simulink model "FAS_Kreuzungswarner_Simulation_V1"  (R2024b)
settings: Solver=FixedStepAuto  StartTime=0.0  StopTime=stoptime  FixedStep=sampletime  RelTol=1e-3
InitFcn:
  | if ~evalin('base', 'exist(''Auswertungsflag'', ''var'')') || evalin('base', 'Auswertungsflag.Value == 0')
  |     Parameterskript;
  |     run('StartGUI');  % explizit ausführen (nicht blockierend!)
  | end
values from neighbouring files (symbols this model uses):
  mEGO = str2double(massEGOInput.String)    [StartGUI.m]
  mFZG = str2double(massFZGInput.String)    [StartGUI.m]
  OeffnungswinkelA = str2double(angleInputA.String)    [StartGUI.m]
  OeffnungswinkelB = Simulink.Parameter    [Auswertung.m]    (also in StartGUI.m = str2double(angleInputB.String))
  P_EGO = str2double(powerEGOInput.String)    [StartGUI.m]
  P_FZG = str2double(powerFZGInput.String)    [StartGUI.m]
  ReichweiteA = str2double(rangeInputA.String)    [StartGUI.m]
  ReichweiteB = str2double(rangeInputB.String)    [StartGUI.m]
  SensorA = sensor1Dropdown.Value    [StartGUI.m]
  SensorB = sensor2Dropdown.Value    [StartGUI.m]
  startPositionEGO = str2double(posEGOInput.String)    [StartGUI.m]
  startPositionFzg = str2double(posFzgInput.String)    [StartGUI.m]
  v_EGO = str2double(velEGOInput.String)    [StartGUI.m]
  v_FZG = str2double(velFZGInput.String)    [StartGUI.m]
  Wetter = weatherDropdown.Value    [StartGUI.m]
  zweitesFzgSwitch = str2double(zweitesFzgInput.String)    [StartGUI.m]
undefined symbols (not defined in the file or in its folder): Airbagzeit, Ausloesezeit, b, dt, g, Haltezeit, l, munass, muschnee, mutrocken, rad_b, rad_l, reifen_dx, reifen_dy, SensorSwitch, startPositionFzg2, xFZG, yEGO
(part 1 of 3)
settings Model: Creator=panic  LastModifiedBy=flori
settings DataIOCC: SaveFormat=StructureWithTime

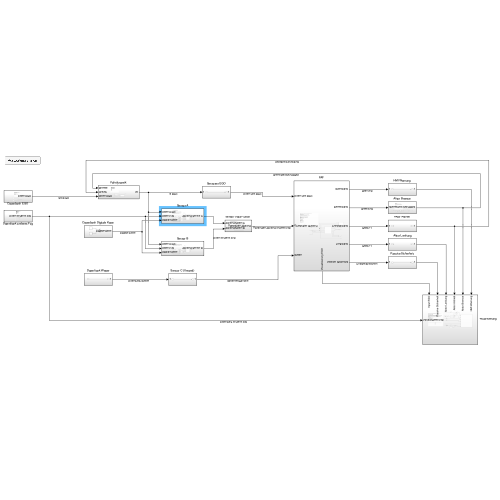
[thumbnail: Simulink's stored preview of the top-level diagram]
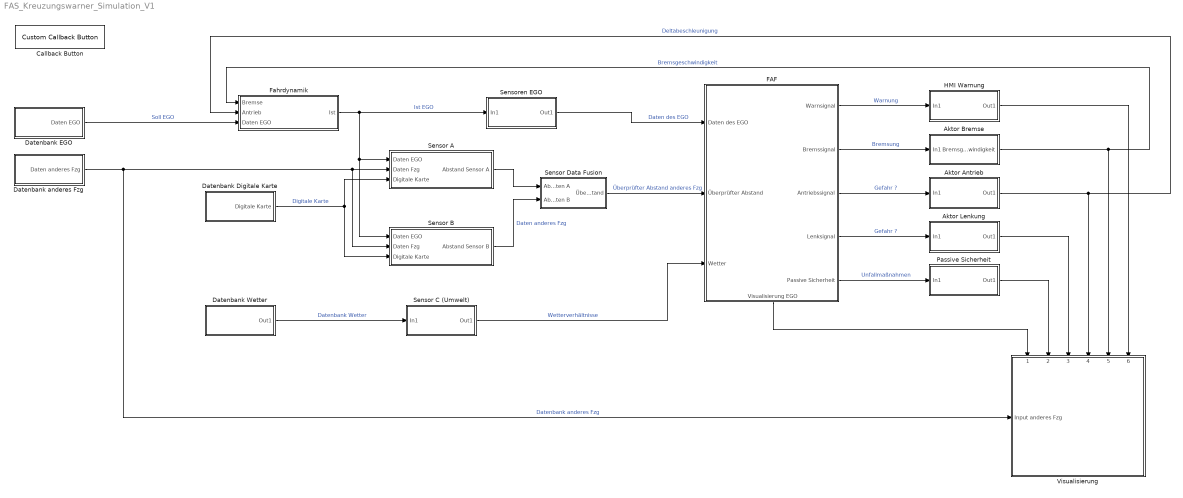
== system FAS_Kreuzungswarner_Simulation_V1 ==
  " Aktor Lenkung" : Subsystem
  Aktor Antrieb : Subsystem
  Aktor Bremse : Subsystem
  Callback Button : CustomCallbackButton  Configuration="{\"components\":[{\"name\":\"BackgroundImageComponent\",\"settings\":{\"image\":{\"size\":[0,0],\"src\":\"default\",\"srcOrientation\":\"Right\"},\"position\":[0,0,1,1]}},{\"name\":\"ButtonStateComponent\",\"settings\":{\"buttonType\":\"momentary\",\"clickFcn\":\"clear all\\nclc\\nassignin('base','Auswertungsbutton',makeParam(1));\\nStartGUI\",\"onValue\":1,\"position\":[0,0,1,1],\"pressDelay\":\"500\",\"pressFcn\":\"\",\"repeatInterval\":\"0\",\"states\":[{\"horizontalAlignment\":\"center\",\"image\":{\"position\":[0,0,1,1],\"size\":[1,1],\"src\":\"default\",\"srcOrientation\":\"Right\"},\"label\":{\"color\":[0,0,0],\"icon\":{\"size\":[0,0],\"src\":\"default\",\"srcOrientation\":\"Right\"},\"iconOffset\":0,\"iconPlacement\":\"left\",\"opacity\":1,\"show\":true,\"text\":{\"content\":\"Auswertung starten\",\"font\":\"Helvetica\"}},\"labelOffset\":[0,0],\"verticalAlignment\":\"middle\"},{\"horizontalAlignment\":\"center\",\"image\":{\"position\":[0,0,1,1],\"size\":[1,1],\"src\":\"default\",\"srcOrientation\":\"Right\"},\"label\":{\"color\":[0.01176470588,0.01176470588,0.01176470588,1],\"icon\":{\"size\":[0,0],\"src\":\"default\",\"srcOrientation\":\"Right\"},\"iconOffset\":0,\"iconPlacement\":\"left\",\"opacity\":1,\"show\":true,\"text\":{\"content\":\"Auswertung starten\",\"font\":\"Helvetica\"}},\"labelOffset\":[0,0],\"verticalAlignment\":\"middle\"},{\"horizontalAlignment\":\"center\",\"image\":{\"position\":[0,0,1,1],\"size\":[1,1],\"src\":\"default\",\"srcOrientation\":\"Right\"},\"label\":{\"color\":[0.01176470588,0.01176470588,0.01176470588,1],\"icon\":{\"size\":[0,0],\"src\":\"default\",\"srcOrientation\":\"Right\"},\"iconOffset\":0,\"iconPlacement\":\"left\",\"opacity\":1,\"show\":true,\"text\":{\"content\":\"Auswertung starten\",\"font\":\"Helvetica\"}},\"labelOffset\":[0,0],\"verticalAlignment\":\"middle\"},{\"horizontalAlignment\":\"center\",\"image\":{\"position\":[0,0,1,1],\"size\":[1,1],\"src\":\"default\",\"srcOrientation\":\"Right\"},\"label\":{\"color\":[0.01176470588,0.01176470588,0.01176470588,1],\"icon\":{\"size\":[0,0],\"src\":\"default\",\"srcOrientation\":\"Right\"},\"iconOffset\":0,\"iconPlacement\":\"left\",\"opacity\":1,\"show\":true,\"text\":{\"content\":\"Auswertung starten\",\"font\":\"Helvetica\"}},\"labelOffset\":[0,0],\"verticalAlignment\":\"middle\"}]}},{\"name\":\"ForegroundImageComponent\",\"settings\":{\"image\":{\"size\":[0,0],\"src\":\"default\",\"srcOrientation\":\"Right\"},\"isForeground\":1,\"position\":[0,0,1,1]}}],\"settings\":{\"BindingType\":\"standalone\",\"backgroundColor\":[244,244,244,1],\"backgroundOffset\":0.2,\"backgroundOpacity\":1,\"fixedAspectRatio\":\"off\",\"foregroundColor\":[0.01176470588,0.01176470588,0.01176470588,1],\"migratedFromLegacy\":true,\"useBackgroundColor\":true,\"variant\":\"callback\",\"version\":\"R2023a\"},\"type\":\"Button\"}"  CustomBackgroundColor="{\"color\":[0.9568627451,0.9568627451,0.9568627451],\"show\":true}"
  Datenbank Digitale Karte : Subsystem
  Datenbank EGO : Subsystem
  Datenbank Wetter : Subsystem
  Datenbank anderes Fzg : Subsystem
  FAF : Subsystem
      settings: PortSchema="{\"entries\":[{\"content\":{\"sides\":[{\"content\":{\"connectorIds\":[\"In1\",\"In2\",\"In3\"]},\"type\":\"ConnectorPlacement.EquallySpacedRectSide\",\"uuid\":\"e9873d16-4c3b-480f-9547-2fedddc84fa2\"},{\"content\":{\"connectorIds\":[\"Out1\",\"Out2\",\"Out3\",\"Out4\",\"Out5\"],\"side\":\"RIGHT\"},\"type\":\"ConnectorPlacement.EquallySpacedRectSide\",\"uuid\":\"f34f386d-1ebd-46c0-87cc-6cf8d85cbe5c\"},{\"content\":{\"side\":\"TOP\"},\"type\":\"ConnectorPlacement.EquallySpacedRectSide\",\"uuid\":\"dae2a922-0ae9-4030-aebb-c1b1f64935ac\"},{\"content\":{\"connectorIds\":[\"Out6\"],\"side\":\"BOTTOM\"},\"type\":\"ConnectorPlacement.EquallySpacedRectSide\",\"uuid\":\"92c182dc-0911-4a88-8c5f-7399a74ff050\"}]},\"type\":\"ConnectorPlacement.EquallySpacedConnector\",\"uuid\":\"9c5e93a9-4ab8-4391-bbf4-9015a537a4fe\"}],\"packageUris\":[\"http://schema.mathworks.com/mf0/Connector/R2020b\"],\"version\":\"1.0\"}"
  Fahrdynamik : Subsystem
  HMI Warnung : Subsystem
  Passive Sicherheit : Subsystem
  Sensor A : Subsystem
  Sensor B : Subsystem
  Sensor C (Umwelt) : Subsystem
  "Sensor Data Fusion " : Subsystem
  Sensoren EGO : Subsystem
  Visualisierung : Subsystem
      settings: PortSchema="{\"entries\":[{\"content\":{\"sides\":[{\"content\":{\"connectorIds\":[\"In1\",\"In2\",\"In3\",\"In4\",\"In5\",\"In6\"]},\"type\":\"ConnectorPlacement.EquallySpacedRectSide\",\"uuid\":\"dd165e45-7e24-4222-b079-fc0a14401503\"},{\"content\":{\"side\":\"RIGHT\"},\"type\":\"ConnectorPlacement.EquallySpacedRectSide\",\"uuid\":\"187c38cf-364e-4c00-8f01-04e514044ebb\"},{\"content\":{\"connectorIds\":[\"In7\"],\"side\":\"TOP\"},\"type\":\"ConnectorPlacement.EquallySpacedRectSide\",\"uuid\":\"80aec09e-8245-4401-9644-d123aeedc7c7\"}]},\"type\":\"ConnectorPlacement.EquallySpacedConnector\",\"uuid\":\"48ae2ddf-e251-4d97-a6a7-fcee22a63fde\"}],\"packageUris\":[\"http://schema.mathworks.com/mf0/Connector/R2020b\"],\"version\":\"1.0\"}"
  wires:
  Fahrdynamik/1(Ist) -> Sensor B/1(Daten EGO), Sensor A/1(Daten EGO), Sensoren EGO/1(In1)  "Ist EGO"
  Sensoren EGO/1(Out1) -> FAF/1(Daten des EGO)  "Daten des EGO"
  Sensor C (Umwelt)/1(Out1) -> FAF/3(Wetter)  "Wetterverhältnisse"
  FAF/3(Antriebssignal) -> Aktor Antrieb/1(In1)  "Gefahr ?"
  FAF/2(Bremssignal) -> Aktor Bremse/1(In1)  "Bremsung"
  FAF/1(Warnsignal) -> HMI Warnung/1(In1)  "Warnung"
  FAF/4(Lenksignal) -> " Aktor Lenkung"/1(In1)  "Gefahr ?"
  FAF/5(Passive Sicherheit) -> Passive Sicherheit/1(In1)  "Unfallmaßnahmen"
  FAF/6(Visualisierung EGO) -> Visualisierung/1(Input EGO)
  Passive Sicherheit/1(Out1) -> Visualisierung/2(Passive Sicherheit)
  " Aktor Lenkung"/1(Out1) -> Visualisierung/3(Aktor Lenkung)
  Aktor Antrieb/1(Out1) -> Visualisierung/4(Aktor Antrieb), Fahrdynamik/2(Antrieb)  "Deltabeschleunigung"
  Aktor Bremse/1(Bremsgeschwindigkeit) -> Visualisierung/5(Aktor Bremse), Fahrdynamik/1(Bremse)  "Bremsgeschwindigkeit"
  HMI Warnung/1(Out1) -> Visualisierung/6(HMI Warnung)
  Datenbank Digitale Karte/1(Digitale Karte) -> Sensor B/3(Digitale Karte), Sensor A/3(Digitale Karte)  "Digitale Karte"
  Datenbank EGO/1(Daten EGO) -> Fahrdynamik/3(Daten EGO)  "Soll EGO"
  Datenbank anderes Fzg/1(Daten anderes Fzg) -> Sensor B/2(Daten Fzg), Sensor A/2(Daten Fzg), Visualisierung/7(Input anderes Fzg)  "Datenbank anderes Fzg"
  Sensor B/1(Abstand Sensor B) -> "Sensor Data Fusion "/2(Abstandsdaten B)  "Daten anderes Fzg"
  Sensor A/1(Abstand Sensor A) -> "Sensor Data Fusion "/1(Abstandsdaten A)
  "Sensor Data Fusion "/1(Überprüfter Abstand) -> FAF/2(Überprüfter Abstand)  "Überprüfter Abstand anderes Fzg"
  Datenbank Wetter/1(Out1) -> Sensor C (Umwelt)/1(In1)  "Datenbank Wetter"

== system FAS_Kreuzungswarner_Simulation_V1/ Aktor Lenkung ==
  In1 : Inport
  Out1 : Outport

== system FAS_Kreuzungswarner_Simulation_V1/Aktor Antrieb ==
  In1 : Inport
  Out1 : Outport

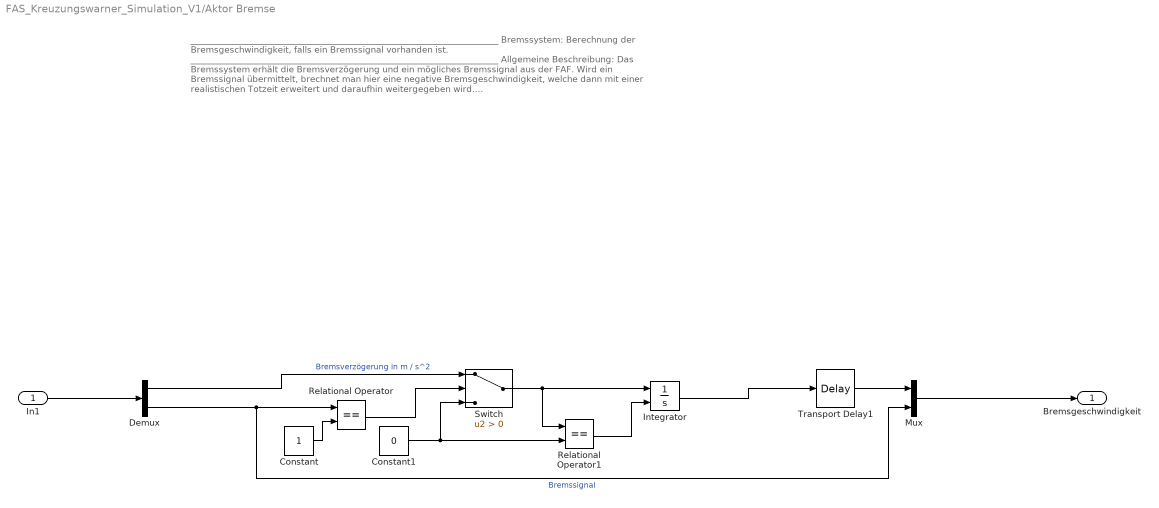
== system FAS_Kreuzungswarner_Simulation_V1/Aktor Bremse ==
  note: _______________________________________________________________________
      | Bremssystem:
      |
      | Berechnung der Bremsgeschwindigkeit, falls ein Bremssignal vorhanden ist.
      | _______________________________________________________________________
      | Allgemeine Beschreibung:
      |
      | Das Bremssystem erhält die Bremsverzögerung und ein mögliches Bremssignal aus
      | der FAF.
      | Wird ein Bremssignal übermittelt, brechnet man hier eine negative Bremsgeschwindigkeit,
      | welche dann mit einer realistischen Totzeit erweitert und daraufhin weitergegeben wird.
      | _______________________________________________________________________
      | Inputs:
      |
      | Das Bremssystem hat zwei Inputs:
      |
      | - Bremsverzögerung [m/s^2]
      | - Bremssignal als 0/1 Signal
      |
      | Outputs:
      |
      | - Berechnete Bremsgeschwindigkeit [m/s]
      | _______________________________________________________________________
  In1 : Inport
  Constant : Constant
  Constant1 : Constant  Value=0
  Demux : Demux  Outputs=2
  Integrator : Integrator  ExternalReset=level
  Mux : Mux  Inputs=2
  Relational Operator : RelationalOperator  Operator===  OutDataTypeStr=boolean  RndMeth=Simplest  InputSameDT=off
  Relational Operator1 : RelationalOperator  Operator===  OutDataTypeStr=boolean  RndMeth=Simplest  InputSameDT=off
  Switch : Switch  Criteria=u2 > Threshold  SaturateOnIntegerOverflow=off  InputSameDT=off
  Transport Delay1 : TransportDelay  DelayTime=0.3
  Bremsgeschwindigkeit : Outport
  wires:
  In1/1 -> Demux/1
  Demux/1 -> Switch/1  "Bremsverzögerung in m / s^2"
  Demux/2 -> Relational Operator/1, Mux/2  "Bremssignal"
  Mux/1 -> Bremsgeschwindigkeit/1
  Constant/1 -> Relational Operator/2
  Relational Operator/1 -> Switch/2
  Relational Operator1/1 -> Integrator/2
  Integrator/1 -> Transport Delay1/1
  Constant1/1 -> Relational Operator1/2, Switch/3
  Switch/1 -> Integrator/1, Relational Operator1/1
  Transport Delay1/1 -> Mux/1

== system FAS_Kreuzungswarner_Simulation_V1/Datenbank Digitale Karte ==
  Mux : Mux  Inputs=2
  xPos Kreuzung : Constant  Value=0
  yPos Kreuzung1 : Constant  Value=0
  Digitale Karte : Outport
  wires:
  Mux/1 -> Digitale Karte/1
  yPos Kreuzung1/1 -> Mux/2
  xPos Kreuzung/1 -> Mux/1

== system FAS_Kreuzungswarner_Simulation_V1/Datenbank EGO ==
  note: _______________________________________________________________________
      | Datenbank EGO:
      |
      | Vorgabe aller Werte die das EGO-Fahrzeug beinhaltet / benötigt.
      | _______________________________________________________________________
      | Allgemeine Beschreibung:
      |
      | Die Werte die das EGO-Fahrzeug erhält werden über das Parameterskript initialisiert und
      | dann über die Eingabe in der GUI angepasst. Daraufhin werden Sie hier in die
      | unterschieldichen Blöcke gespeichert.
      | Die Geschwindigkeit wird nach der Eingabe in m/s umgerechnet.
      | _______________________________________________________________________
      | Inputs:
      |
      | Die Datenbank des EGOs beinhaltet drei Werte:
      |
      | - Motorleistung_EGO [kW]
      | - Fahrzeugmasse_EGO [kg]
      | - Geschwindikeit_EGO [km/h]
      |
      | Outputs:
      |
      | Diese Werte werden dann an die Fahrdynamik weitergeleitet.
      | ______________________________________________________________________
  Fahrzeugmasse in kg : Constant  Value=mEGO
  Gain : Gain  Gain=1/3.6
  Geschwindigkeit km/h : Constant  Value=v_EGO
  Motorleistung in kW : Constant  Value=P_EGO
  Mux : Mux  Inputs=3
  Daten EGO : Outport
  wires:
  Fahrzeugmasse in kg/1 -> Mux/2
  Motorleistung in kW/1 -> Mux/1
  Mux/1 -> Daten EGO/1
  Geschwindigkeit km/h/1 -> Gain/1
  Gain/1 -> Mux/3  "GeschwindigkeitEGO in m/s"

== system FAS_Kreuzungswarner_Simulation_V1/Datenbank Wetter ==
  Regen : Constant  Value=Wetter
  Out1 : Outport
  wires:
  Regen/1 -> Out1/1

== system FAS_Kreuzungswarner_Simulation_V1/Datenbank anderes Fzg ==
  note: _______________________________________________________________________
      | Datenbank anderes Fahrzeug:
      |
      | Vorgabe aller Werte die die anderen Fahrzeuge beinhalten / benötigen.
      | _______________________________________________________________________
      | Allgemeine Beschreibung:
      |
      | Die Werte die das andere Fahrzeug erhält werden über das Parameterskript initialisiert und
      | dann über die Eingabe in der GUI angepasst. Daraufhin werden Sie hier in die
      | unterschiedlichen Blöcke gespeichert.
      | Zusätzlich werden auch hier nochmals die Werte des EGO-Fahrzeugs verwendet (diese werden für das Szenario mit dem vorrausfahrenden Fahrzeug (zweites FZG) benötigt).
      | Die Geschwindigkeiten werden nach der Eingabe in m/s umgerechnet.
      | _______________________________________________________________________
      | Inputs:
      |
      | Die Datenbank der anderen Fahrzeuge beinhaltet folgende Werte:
      |
      | - Motorleistung des anderen Fahrzeugs [kW]
      | - Fahrzeugmasse des anderen Fahrzeugs [kg]
      | - Geschwindigkeit des anderen Fahrzeugs [km/h]
      |
      | - Motorleistung_EGO [kW]
      | - Fahrzeugmasse_EGO [kg]
      | - Geschwindikeit_EGO [km/h]
      |
      | Outputs:
      |
      | Diese Werte werden dann teilweise an die Sensoren (A und B), aber auch an die
      | Visualisierung weitergeleitet.
      | ______________________________________________________________________
  Fahrzeugmasse in kg : Constant  Value=mFZG
  Fahrzeugmasse in kg1 : Constant  Value=mEGO
  Gain : Gain  Gain=1/3.6
  Gain1 : Gain  Gain=1/3.6
  Geschwindigkeit km/h : Constant  Value=v_FZG
  Geschwindigkeit km/h1 : Constant  Value=v_EGO
  Motorleistung in kW : Constant  Value=P_FZG
  Motorleistung in kW1 : Constant  Value=P_EGO
  Mux : Mux  Inputs=6
  Daten anderes Fzg : Outport
  wires:
  Fahrzeugmasse in kg/1 -> Mux/2
  Motorleistung in kW/1 -> Mux/1
  Geschwindigkeit km/h/1 -> Gain/1
  Mux/1 -> Daten anderes Fzg/1
  Gain/1 -> Mux/3
  Geschwindigkeit km/h1/1 -> Gain1/1
  Fahrzeugmasse in kg1/1 -> Mux/5
  Gain1/1 -> Mux/6
  Motorleistung in kW1/1 -> Mux/4

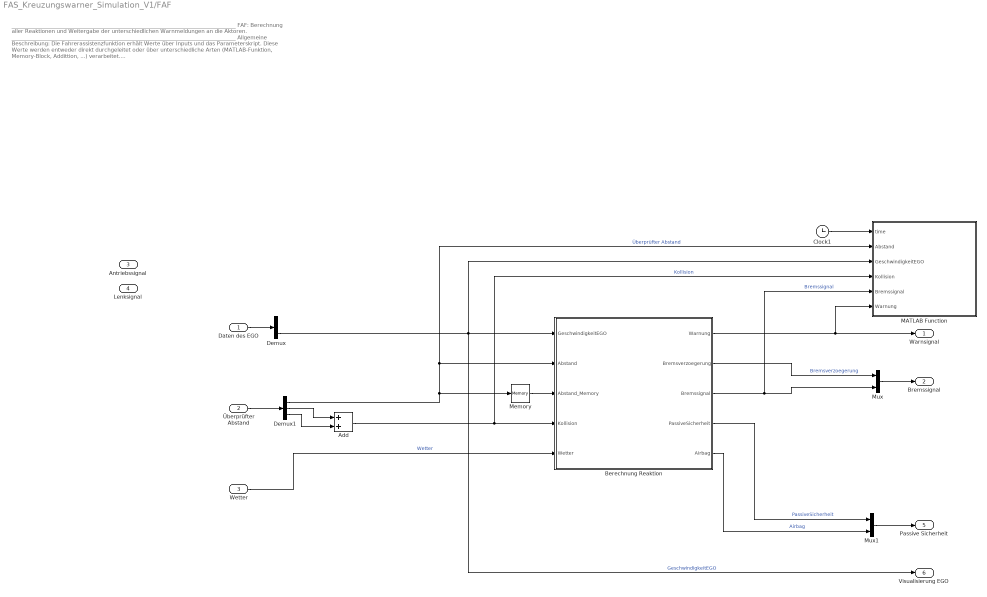
== system FAS_Kreuzungswarner_Simulation_V1/FAF ==
  note: ____________________________________________________________________________________
      | FAF:
      |
      | Berechnung aller Reaktionen und Weitergabe der unterschiedlichen Warnmeldungen an die Aktoren.
      | ____________________________________________________________________________________
      | Allgemeine Beschreibung:
      |
      | Die Fahrerassistenzfunktion erhält Werte über Inputs und das Parameterskript.
      | Diese Werte werden entweder direkt durchgeleitet oder über unterschiedliche Arten
      | (MATLAB-Funktion, Memory-Block, Addittion, ...) verarbeitet.
      | ____________________________________________________________________________________
      | Inputs:
      |
      | Die FAF beinhaltet aktive, während der Simulation veränderliche, Inputs:
      |
      | - Geschwindikeit_EGO [m/s]
      | - Abstand [m]
      | - Abstand_Memory [m] (= Abstand des vorherigen Simulationsschritts)
      | - Kollision als 0/1 Signal (wenn Kollision = 1, Fahrzeuge treffen sich)
      | - Wetter (Trocken, Regen und Schnee)
      |
      | Outputs:
      |
      | - Warnung als 0/1 Signal
      | - Bremsverzögerung in m/s^2
      | - Bremssignal als 0/1 Signal
      | - Passive Sicherheit als 0/1 Signal
      | - Airbag als 0/1 Signal
      |
      | Reserve
      | - Antriebssignal für spätere Projekte
      |
      | - Lenksignal für spätere Projekte
      |
      | _______________________________________________________________________
  Daten des EGO : Inport
  Überprüfter Abstand : Inport  Port=2
  Wetter : Inport  Port=3
  Add : Sum
  Berechnung Reaktion : MATLAB Function  TreatAsAtomicUnit=on
  Clock1 : Clock
  Demux : Demux  Outputs=3
  Demux1 : Demux  Outputs=3
  MATLAB Function : MATLAB Function  TreatAsAtomicUnit=on  SystemSampleTime=sampletime
  Memory : Memory  InheritSampleTime=on
  Mux : Mux  Inputs=2
  Mux1 : Mux  Inputs=2
  Warnsignal : Outport
  Bremssignal : Outport  Port=2
  Antriebssignal : Outport  Port=3
  Lenksignal : Outport  Port=4
  Passive Sicherheit : Outport  Port=5
  Visualisierung EGO : Outport  Port=6
  wires:
  Berechnung Reaktion/4(PassiveSicherheit) -> Mux1/1  "PassiveSicherheit"
  Berechnung Reaktion/1(Warnung) -> Warnsignal/1, MATLAB Function/6(Warnung)
  Daten des EGO/1 -> Demux/1
  Demux/3 -> Berechnung Reaktion/1(GeschwindigkeitEGO), Visualisierung EGO/1, MATLAB Function/3(GeschwindigkeitEGO)  "GeschwindigkeitEGO"
  Wetter/1 -> Berechnung Reaktion/5(Wetter)  "Wetter"
  Berechnung Reaktion/3(Bremssignal) -> MATLAB Function/5(Bremssignal), Mux/2  "Bremssignal"
  Mux/1 -> Bremssignal/1
  Berechnung Reaktion/2(Bremsverzoegerung) -> Mux/1  "Bremsverzoegerung"
  Memory/1 -> Berechnung Reaktion/3(Abstand_Memory)
  Berechnung Reaktion/5(Airbag) -> Mux1/2  "Airbag"
  Mux1/1 -> Passive Sicherheit/1
  Überprüfter Abstand/1 -> Demux1/1
  Demux1/1 -> Berechnung Reaktion/2(Abstand), MATLAB Function/2(Abstand), Memory/1  "Überprüfter Abstand"
  Demux1/2 -> Add/1
  Demux1/3 -> Add/2
  Add/1 -> Berechnung Reaktion/4(Kollision), MATLAB Function/4(Kollision)  "Kollision"
  Clock1/1 -> MATLAB Function/1(time)

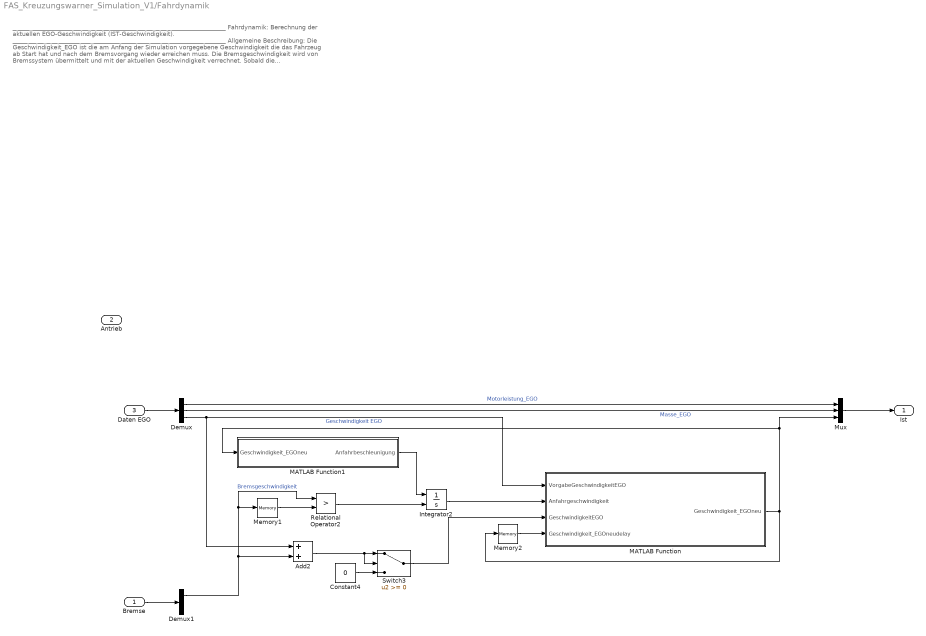
== system FAS_Kreuzungswarner_Simulation_V1/Fahrdynamik ==
  note: _______________________________________________________________________
      | Fahrdynamik:
      |
      | Berechnung der aktuellen EGO-Geschwindigkeit (IST-Geschwindigkeit).
      | _______________________________________________________________________
      | Allgemeine Beschreibung:
      |
      | Die Geschwindigkeit_EGO ist die am Anfang der Simulation vorgegebene
      | Geschwindigkeit die das Fahrzeug ab Start hat und nach dem Bremsvorgang wieder
      | erreichen muss. Die Bremsgeschwindigkeit wird von Bremssystem übermittelt und mit
      | der aktuellen Geschwindigkeit verrechnet.
      | Sobald die Bremsgeschwindigkeit größer wird als im Simulationsschritt zuvor, wird der
      | Integrator zurückgesetzt. Dieser Integrator berechnet die Geschwindigkeit durch
      | Integrieren der aktuellen, abhängig von Motorleistung, Reibung und Schlupf,
      | berrechneten Anfahrbeschleunigung. Diese Geschwindigkeit wird dann mit der
      | momentanen Geschwindigkeit des EGOs verrechnet und dadurch wird ein realistisches
      | Anfahren simuliert.
      | _______________________________________________________________________
      | Inputs:
      |
      | Die Fahrdynamik beinhaltet aktive, während der Simulation veränderliche, Inputs:
      |
      | - Bremsgeschwindigkeit [m/s]
      | - Motorleistung_EGO [kW]
      | - Masse_EGO [kg]
      | - Geschwindigkeit_EGO [m/s]
      |
      | Outputs:
      |
      | - Motorleistung_EGO [kW]
      | - Masse_EGO [kg]
      | - Geschwindigkeit_EGOneu [m/s]
      |
      | Reserve
      | - Antrieb für spätere Projekte
      |
      | _______________________________________________________________________
  Bremse : Inport
  Antrieb : Inport  Port=2
  Daten EGO : Inport  Port=3
  Add2 : Sum
  Constant4 : Constant  Value=0
  Demux : Demux  Outputs=3
  Demux1 : Demux  Outputs=2
  Integrator2 : Integrator  ExternalReset=rising
  MATLAB Function : MATLAB Function  TreatAsAtomicUnit=on  SystemSampleTime=sampletime
  MATLAB Function1 : MATLAB Function  TreatAsAtomicUnit=on
  Memory1 : Memory  InheritSampleTime=on
  Memory2 : Memory  InheritSampleTime=on
  Mux : Mux  Inputs=3
  Relational Operator2 : RelationalOperator  Operator=>  OutDataTypeStr=boolean  RndMeth=Simplest  InputSameDT=off
  Switch3 : Switch  SaturateOnIntegerOverflow=off  InputSameDT=off
  Ist : Outport
  wires:
  Daten EGO/1 -> Demux/1
  Mux/1 -> Ist/1
  Demux/1 -> Mux/1  "Motorleistung_EGO"
  Demux/2 -> Mux/2  "Masse_EGO"
  Bremse/1 -> Demux1/1
  Demux/3 -> Add2/1, MATLAB Function/1(VorgabeGeschwindigkeitEGO)  "Geschwindigkeit EGO"
  Add2/1 -> Switch3/2, Switch3/1
  Constant4/1 -> Switch3/3
  Memory1/1 -> Relational Operator2/2
  Demux1/1 -> Relational Operator2/1, Memory1/1, Add2/2  "Bremsgeschwindigkeit"
  Relational Operator2/1 -> Integrator2/2
  Integrator2/1 -> MATLAB Function/2(Anfahrgeschwindigkeit)
  Switch3/1 -> MATLAB Function/3(GeschwindigkeitEGO)
  Memory2/1 -> MATLAB Function/4(Geschwindigkeit_EGOneudelay)
  MATLAB Function/1(Geschwindigkeit_EGOneu) -> Memory2/1, Mux/3, MATLAB Function1/1(Geschwindigkeit_EGOneu)
  MATLAB Function1/1(Anfahrbeschleunigung) -> Integrator2/1

== system FAS_Kreuzungswarner_Simulation_V1/HMI Warnung ==
  In1 : Inport
  Out1 : Outport
  wires:
  In1/1 -> Out1/1

== system FAS_Kreuzungswarner_Simulation_V1/Passive Sicherheit ==
  In1 : Inport
  Out1 : Outport
  wires:
  In1/1 -> Out1/1

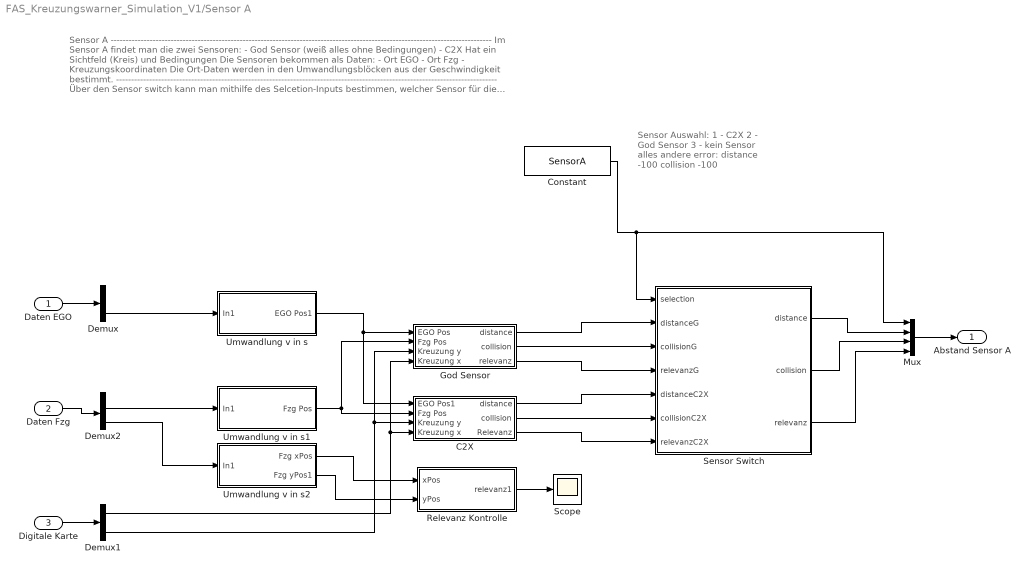
== system FAS_Kreuzungswarner_Simulation_V1/Sensor A ==
  note: Sensor A
      | -------------------------------------------------------------------------------------------------------------------------------
      | Im Sensor A findet man die zwei Sensoren:
      | - God Sensor (weiß alles ohne Bedingungen)
      | - C2X Hat ein Sichtfeld (Kreis) und Bedingungen
      | Die Sensoren bekommen als Daten:
      | - Ort EGO
      | - Ort Fzg
      | - Kreuzungskoordinaten
      | Die Ort-Daten werden in den Umwandlungsblöcken aus der Geschwindigkeit bestimmt.
      | -------------------------------------------------------------------------------------------------------------------------------
      | Über den Sensor switch kann man mithilfe des Selcetion-Inputs bestimmen, welcher Sensor für die aktuelle Simulation verwendet wird. Der Const.-Block "Sensor A" wird über die GUI gesteuert.
      | -------------------------------------------------------------------------------------------------------------------------------
      | Die Relevanz Kontrolle prüft ob ein weiteres Fzg sich auf der gleichen Achse wie das EGO befindet. Dieser Output wird stand jetzt aber noch nicht weiterverwendet
  note: Sensor Auswahl:
      | 1 - C2X
      | 2 - God Sensor
      | 3 - kein Sensor
      | alles andere error:
      | distance -100
      | collision -100
  Daten EGO : Inport
  Daten Fzg : Inport  Port=2
  Digitale Karte : Inport  Port=3
  C2X : Subsystem
  Constant : Constant  Value=SensorA
  Demux : Demux  Outputs=3
  Demux1 : Demux  Outputs=2
  Demux2 : Demux  Outputs=6
  God Sensor : Subsystem
  Mux : Mux
  Relevanz Kontrolle : Subsystem
  Scope : Scope
  Sensor Switch : MATLAB Function  TreatAsAtomicUnit=on
  Umwandlung v in s : Subsystem
  Umwandlung v in s1 : Subsystem
  Umwandlung v in s2 : Subsystem
  Abstand Sensor A : Outport
  wires:
  Daten EGO/1 -> Demux/1
  Demux/3 -> Umwandlung v in s/1(In1)
  Digitale Karte/1 -> Demux1/1
  Demux1/2 -> God Sensor/3(Kreuzung y), C2X/3(Kreuzung y)
  Umwandlung v in s/1(EGO Pos1) -> C2X/1(EGO Pos1), God Sensor/1(EGO Pos)
  Daten Fzg/1 -> Demux2/1
  Demux2/3 -> Umwandlung v in s1/1(In1)
  Constant/1 -> Mux/1, Sensor Switch/1(selection)
  C2X/1(distance) -> Sensor Switch/5(distanceC2X)
  C2X/2(collision) -> Sensor Switch/6(collisionC2X)
  Sensor Switch/1(distance) -> Mux/2
  Sensor Switch/2(collision) -> Mux/3
  God Sensor/1(distance) -> Sensor Switch/2(distanceG)
  God Sensor/2(collision) -> Sensor Switch/3(collisionG)
  God Sensor/3(relevanz) -> Sensor Switch/4(relevanzG)
  Umwandlung v in s1/1(Fzg Pos) -> God Sensor/2(Fzg Pos), C2X/2(Fzg Pos)
  Sensor Switch/3(relevanz) -> Mux/4
  Mux/1 -> Abstand Sensor A/1
  C2X/3(Relevanz) -> Sensor Switch/7(relevanzC2X)
  Demux2/6 -> Umwandlung v in s2/1(In1)
  Demux1/1 -> God Sensor/4(Kreuzung x), C2X/4(Kreuzung x)
  Umwandlung v in s2/1(Fzg xPos) -> Relevanz Kontrolle/1(xPos)
  Umwandlung v in s2/2(Fzg yPos1) -> Relevanz Kontrolle/2(yPos)
  Relevanz Kontrolle/1(relevanz1) -> Scope/1

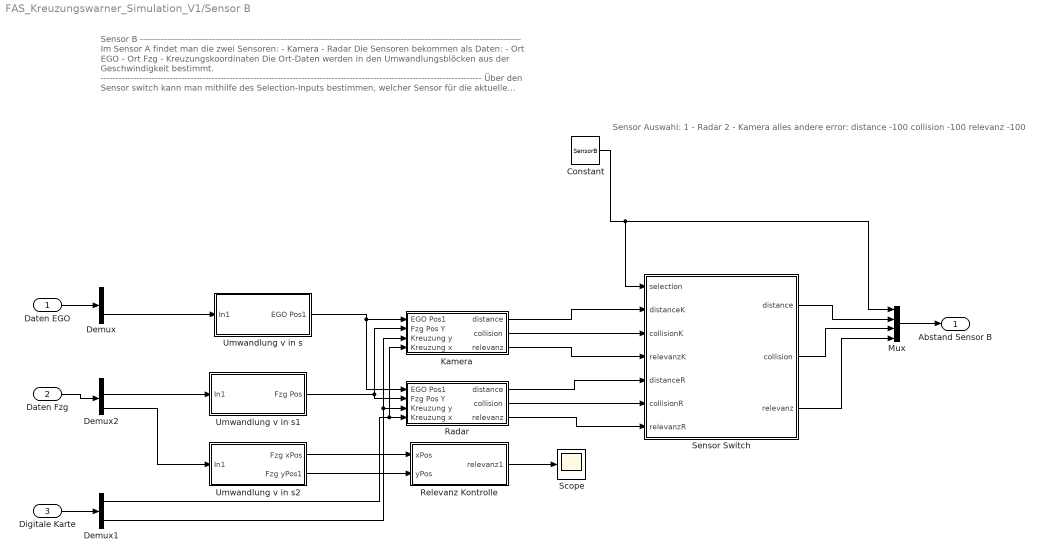
== system FAS_Kreuzungswarner_Simulation_V1/Sensor B ==
  note: Sensor Auswahl:
      | 1 - Radar
      | 2 - Kamera
      | alles andere error:
      | distance -100
      | collision -100
      | relevanz -100
  note: Sensor B
      | -------------------------------------------------------------------------------------------------------------------------------
      | Im Sensor A findet man die zwei Sensoren:
      | - Kamera
      | - Radar
      | Die Sensoren bekommen als Daten:
      | - Ort EGO
      | - Ort Fzg
      | - Kreuzungskoordinaten
      | Die Ort-Daten werden in den Umwandlungsblöcken aus der Geschwindigkeit bestimmt.
      | -------------------------------------------------------------------------------------------------------------------------------
      | Über den Sensor switch kann man mithilfe des Selection-Inputs bestimmen, welcher Sensor für die aktuelle Simulation verwendet wird. Der Const.-Block "Sensor A" wird über die GUI gesteuert.
      | -------------------------------------------------------------------------------------------------------------------------------
      | Die Relevanz Kontrolle prüft ob ein weiteres Fzg sich auf der gleichen Achse wie das EGO befindet. Dieser Output wird stand jetzt aber noch nicht weiterverwendet
  Daten EGO : Inport
  Daten Fzg : Inport  Port=2
  Digitale Karte : Inport  Port=3
  Constant : Constant  Value=SensorB
  Demux : Demux  Outputs=3
  Demux1 : Demux  Outputs=2
  Demux2 : Demux  Outputs=6
  Kamera : Subsystem
  Mux : Mux
  Radar : Subsystem
  Relevanz Kontrolle : Subsystem
  Scope : Scope
  Sensor Switch : MATLAB Function  TreatAsAtomicUnit=on
  Umwandlung v in s : Subsystem
  Umwandlung v in s1 : Subsystem
  Umwandlung v in s2 : Subsystem
  Abstand Sensor B : Outport
  wires:
  Daten EGO/1 -> Demux/1
  Demux/3 -> Umwandlung v in s/1(In1)
  Digitale Karte/1 -> Demux1/1
  Demux1/2 -> Kamera/3(Kreuzung y), Radar/3(Kreuzung y)
  Umwandlung v in s/1(EGO Pos1) -> Radar/1(EGO Pos1), Kamera/1(EGO Pos1)
  Daten Fzg/1 -> Demux2/1
  Demux2/3 -> Umwandlung v in s1/1(In1)
  Constant/1 -> Mux/1, Sensor Switch/1(selection)
  Mux/1 -> Abstand Sensor B/1
  Sensor Switch/1(distance) -> Mux/2
  Sensor Switch/2(collision) -> Mux/3
  Umwandlung v in s1/1(Fzg Pos) -> Radar/2(Fzg Pos Y), Kamera/2(Fzg Pos Y)
  Sensor Switch/3(relevanz) -> Mux/4
  Kamera/1(distance) -> Sensor Switch/2(distanceK)
  Kamera/2(collision) -> Sensor Switch/3(collisionK)
  Kamera/3(relevanz) -> Sensor Switch/4(relevanzK)
  Radar/1(distance) -> Sensor Switch/5(distanceR)
  Radar/2(collision) -> Sensor Switch/6(collisionR)
  Demux1/1 -> Kamera/4(Kreuzung x), Radar/4(Kreuzung x)
  Radar/3(relevanz) -> Sensor Switch/7(relevanzR)
  Demux2/6 -> Umwandlung v in s2/1(In1)
  Umwandlung v in s2/1(Fzg xPos) -> Relevanz Kontrolle/1(xPos)
  Umwandlung v in s2/2(Fzg yPos1) -> Relevanz Kontrolle/2(yPos)
  Relevanz Kontrolle/1(relevanz1) -> Scope/1

== system FAS_Kreuzungswarner_Simulation_V1/Sensor C (Umwelt) ==
  In1 : Inport
  Out1 : Outport
  wires:
  In1/1 -> Out1/1

== system FAS_Kreuzungswarner_Simulation_V1/Sensor Data Fusion  ==
  note: Sensor Data Fusion
      | ------------------------------------------------------------------------------------------------
      | In der Sensor Data Fusion werden die Daten Relevanz und Abstand der
      | Sensoren A und B miteinander verbunden (Siehe Logik in den Blöcken).
      | Als Output erhält man einen überprüften Abstand.
  Abstandsdaten A : Inport
  Abstandsdaten B : Inport  Port=2
  Demux : Demux
  Demux1 : Demux
  Mux : Mux  Inputs=3
  Scope : Scope  NumInputPorts=8
  Verarbeitung Abstand : MATLAB Function  TreatAsAtomicUnit=on
  Verarbeitung Relevanz : MATLAB Function  TreatAsAtomicUnit=on
  Zusammenführung : MATLAB Function  TreatAsAtomicUnit=on
  Überprüfter Abstand : Outport
  wires:
  Abstandsdaten B/1 -> Demux/1
  Abstandsdaten A/1 -> Demux1/1
  Demux1/4 -> Scope/5, Verarbeitung Relevanz/1(relevanzA)  "Relevanz A"
  Demux1/2 -> Scope/1, Verarbeitung Abstand/1(distanceA)  "Abstand A"
  Demux/2 -> Scope/2, Verarbeitung Abstand/2(distanceB)  "Abstand B"
  Demux/4 -> Scope/3, Verarbeitung Relevanz/2(relevanzB)  "Relevanz B"
  Zusammenführung/1(distanceO) -> Mux/1, Scope/6
  Verarbeitung Abstand/1(distance) -> Scope/8, Zusammenführung/1(distanceI)
  Verarbeitung Relevanz/1(relevanz) -> Scope/4, Zusammenführung/2(relevanz)
  Mux/1 -> Überprüfter Abstand/1
  Demux/3 -> Scope/7, Mux/3  "Kollisionsdaten für die Auswertung"
  Demux1/3 -> Mux/2

== system FAS_Kreuzungswarner_Simulation_V1/Sensoren EGO ==
  In1 : Inport
  Out1 : Outport
  wires:
  In1/1 -> Out1/1

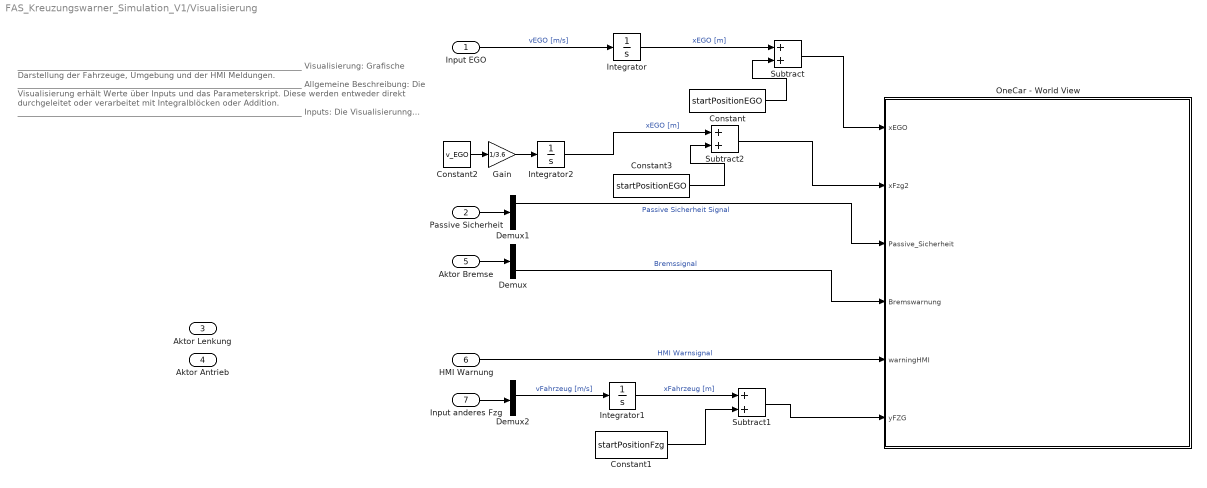
== system FAS_Kreuzungswarner_Simulation_V1/Visualisierung ==
  note: _______________________________________________________________________
      | Visualisierung:
      |
      | Grafische Darstellung der Fahrzeuge, Umgebung und der HMI Meldungen.
      | _______________________________________________________________________
      | Allgemeine Beschreibung:
      |
      | Die Visualisierung erhält Werte über Inputs und das Parameterskript.
      | Diese werden entweder direkt durchgeleitet oder verarbeitet mit Integralblöcken oder Addition.
      | _______________________________________________________________________
      | Inputs:
      |
      | Die Visualisierunng beinhaltet aktive, während der Simulation veränderliche, Inputs:
      |
      | - Input EGO [m/s]
      | - Passive Sicherheit als 0/1 Signal
      | - Aktor Bremse als 0/1 Signal
      | - HMI Warnung als 0/1 Signal
      |
      | Reserve:
      | - Aktor Lenkung für spätere Projekte
      |
      | - Aktor Antrieb für spätere Projekte
      |
      | _______________________________________________________________________
  Input EGO : Inport
  Passive Sicherheit : Inport  Port=2
  Aktor Lenkung : Inport  Port=3
  Aktor Antrieb : Inport  Port=4
  Aktor Bremse : Inport  Port=5
  HMI Warnung : Inport  Port=6
  Input anderes Fzg : Inport  Port=7
  Constant : Constant  Value=startPositionEGO
  Constant1 : Constant  Value=startPositionFzg
  Constant2 : Constant  Value=v_EGO
  Constant3 : Constant  Value=startPositionEGO
  Demux : Demux  Outputs=2
  Demux1 : Demux  Outputs=2
  Demux2 : Demux  Outputs=6
  Gain : Gain  Gain=1/3.6
  Integrator : Integrator
  Integrator1 : Integrator
  Integrator2 : Integrator
  OneCar - World View : MATLAB Function  TreatAsAtomicUnit=on
  Subtract : Sum
  Subtract1 : Sum
  Subtract2 : Sum
  wires:
  Input EGO/1 -> Integrator/1  "vEGO [m/s]"
  Integrator/1 -> Subtract/1  "xEGO [m]"
  Subtract/1 -> OneCar - World View/1(xEGO)
  Constant/1 -> Subtract/2
  Aktor Bremse/1 -> Demux/1
  Passive Sicherheit/1 -> Demux1/1
  Constant1/1 -> Subtract1/2
  Integrator1/1 -> Subtract1/1  "xFahrzeug [m]"
  Subtract1/1 -> OneCar - World View/6(yFZG)
  Input anderes Fzg/1 -> Demux2/1
  Demux2/3 -> Integrator1/1  "vFahrzeug [m/s]"
  Demux1/1 -> OneCar - World View/3(Passive_Sicherheit)  "Passive Sicherheit Signal"
  HMI Warnung/1 -> OneCar - World View/5(warningHMI)  "HMI Warnsignal"
  Demux/2 -> OneCar - World View/4(Bremswarnung)  "Bremssignal"
  Constant2/1 -> Gain/1
  Constant3/1 -> Subtract2/2
  Integrator2/1 -> Subtract2/1  "xEGO [m]"
  Subtract2/1 -> OneCar - World View/2(xFzg2)
  Gain/1 -> Integrator2/1

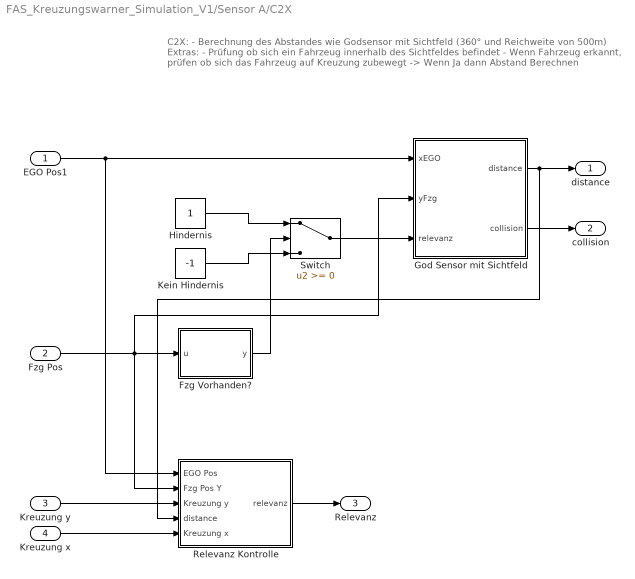
== system FAS_Kreuzungswarner_Simulation_V1/Sensor A/C2X ==
  note: C2X:
      | - Berechnung des Abstandes wie Godsensor mit Sichtfeld (360° und Reichweite von 500m)
      | Extras:
      | - Prüfung ob sich ein Fahrzeug innerhalb des Sichtfeldes befindet
      | - Wenn Fahrzeug erkannt, prüfen ob sich das Fahrzeug auf Kreuzung zubewegt
      | -> Wenn Ja dann Abstand Berechnen
  EGO Pos1 : Inport
  Fzg Pos : Inport  Port=2
  Kreuzung y : Inport  Port=3
  Kreuzung x : Inport  Port=4
  Fzg Vorhanden? : MATLAB Function  TreatAsAtomicUnit=on
  God Sensor mit Sichtfeld : MATLAB Function  TreatAsAtomicUnit=on
  Hindernis : Constant
  Kein Hindernis : Constant  Value=-1
  Relevanz Kontrolle : Subsystem
  Switch : Switch  SaturateOnIntegerOverflow=off  InputSameDT=off
  distance : Outport
  collision : Outport  Port=2
  Relevanz : Outport  Port=3
  wires:
  Fzg Pos/1 -> Relevanz Kontrolle/2(Fzg Pos Y), God Sensor mit Sichtfeld/2(yFzg), Fzg Vorhanden?/1(u)
  Kein Hindernis/1 -> Switch/3
  Switch/1 -> God Sensor mit Sichtfeld/3(relevanz)
  Hindernis/1 -> Switch/1
  Fzg Vorhanden?/1(y) -> Switch/2
  EGO Pos1/1 -> Relevanz Kontrolle/1(EGO Pos), God Sensor mit Sichtfeld/1(xEGO)
  God Sensor mit Sichtfeld/2(collision) -> collision/1
  God Sensor mit Sichtfeld/1(distance) -> Relevanz Kontrolle/4(distance), distance/1
  Relevanz Kontrolle/1(relevanz) -> Relevanz/1
  Kreuzung y/1 -> Relevanz Kontrolle/3(Kreuzung y)
  Kreuzung x/1 -> Relevanz Kontrolle/5(Kreuzung x)

== system FAS_Kreuzungswarner_Simulation_V1/Sensor A/God Sensor ==
  note: God Sensor
      | -----------------------------------------------------------------------------------------------------------
      | God Sensor Funktionsblock mit der allgemeinen Relevanz Kontrolle
      | -----------------------------------------------------------------------------------------------------------
      | Der Godsensor Funktionsblock nimmt die Bewegungsrichtung des EGOs und
      | Fzgs als Input und gibt Daten einer Distanz und Kollisionserkennung zurück.
      | -----------------------------------------------------------------------------------------------------------
      | Die Relevanz Kontrolle prüft, wie Relevant das Erkannte Fzg ist
  EGO Pos : Inport
  Fzg Pos : Inport  Port=2
  Kreuzung y : Inport  Port=3
  Kreuzung x : Inport  Port=4
  God Sensor : MATLAB Function  TreatAsAtomicUnit=on
  Relevanz Kontrolle : Subsystem
  distance : Outport
  collision : Outport  Port=2
  relevanz : Outport  Port=3
  wires:
  Fzg Pos/1 -> God Sensor/2(yFzg), Relevanz Kontrolle/2(Fzg Pos Y)
  EGO Pos/1 -> Relevanz Kontrolle/1(EGO Pos), God Sensor/1(xEGO)
  God Sensor/2(collision) -> collision/1
  God Sensor/1(distance) -> Relevanz Kontrolle/4(distance), distance/1
  Relevanz Kontrolle/1(relevanz) -> relevanz/1
  Kreuzung y/1 -> Relevanz Kontrolle/3(Kreuzung y)
  Kreuzung x/1 -> Relevanz Kontrolle/5(Kreuzung x)

== system FAS_Kreuzungswarner_Simulation_V1/Sensor A/Relevanz Kontrolle ==
  note: Gibt eine 1 aus wenn Fzg auf y Achse Fährt
      | Gibt eine -1 aus wenn Fzg auf x Achse Fährt
  xPos : Inport
  yPos : Inport  Port=2
  Bewegungs-Achse Fzg1 : MATLAB Function  TreatAsAtomicUnit=on
  Const -1 : Constant  Value=-1
  Const 1 : Constant
  Switch1 : Switch  Criteria=u2 > Threshold  Threshold=1  SaturateOnIntegerOverflow=off  InputSameDT=off
  Unit Delay4 : UnitDelay  SampleTime=-1  HasFrameUpgradeWarning=on
  Unit Delay5 : UnitDelay  SampleTime=-1  HasFrameUpgradeWarning=on
  relevanz1 : Outport
  wires:
  Const -1/1 -> Switch1/3
  Unit Delay4/1 -> Bewegungs-Achse Fzg1/2(xFzg_prev)
  yPos/1 -> Unit Delay5/1, Bewegungs-Achse Fzg1/3(yFzg)
  Unit Delay5/1 -> Bewegungs-Achse Fzg1/4(yFzg_prev)
  xPos/1 -> Unit Delay4/1, Bewegungs-Achse Fzg1/1(xFzg)
  Const 1/1 -> Switch1/1
  Switch1/1 -> relevanz1/1
  Bewegungs-Achse Fzg1/1(bewegung) -> Switch1/2

== system FAS_Kreuzungswarner_Simulation_V1/Sensor A/Umwandlung v in s ==
  note: Integrieren der Geschwindigkeit, um auf die Position zu kommen.
      | Davon wird dann die Startpos hinzugerechnet
  In1 : Inport
  Add : Sum
  Constant : Constant  Value=startPositionEGO
  Integrator : Integrator
  EGO Pos1 : Outport
  wires:
  Add/1 -> EGO Pos1/1
  Constant/1 -> Add/2
  Integrator/1 -> Add/1
  In1/1 -> Integrator/1

== system FAS_Kreuzungswarner_Simulation_V1/Sensor A/Umwandlung v in s1 ==
  note: Integrieren der Geschwindigkeit, um auf die Position zu kommen.
      | Davon wird dann die Startpos hinzugerechnet
  In1 : Inport
  Add : Sum
  Constant : Constant  Value=startPositionFzg
  Integrator : Integrator
  Fzg Pos : Outport
  wires:
  Add/1 -> Fzg Pos/1
  Constant/1 -> Add/2
  Integrator/1 -> Add/1
  In1/1 -> Integrator/1

== system FAS_Kreuzungswarner_Simulation_V1/Sensor A/Umwandlung v in s2 ==
  note: Integrieren der Geschwindigkeit, um auf die Position zu kommen.
      | Davon wird dann die Startpos hinzugerechnet
  In1 : Inport
  Add : Sum
  Constant : Constant  Value=startPositionFzg2
  Constant1 : Constant  Value=yEGO
  Integrator : Integrator
  Fzg xPos : Outport
  Fzg yPos1 : Outport  Port=2
  wires:
  Add/1 -> Fzg xPos/1
  Constant/1 -> Add/2
  Integrator/1 -> Add/1
  In1/1 -> Integrator/1
  Constant1/1 -> Fzg yPos1/1

== system FAS_Kreuzungswarner_Simulation_V1/Sensor B/Kamera ==
  note: Kamera
      | -----------------------------------------------------------------------------------------------------------
      | God Sensor mit Sichtfeld Funktionsblock mit der allgemeinen Relevanz Kontrolle
      | -----------------------------------------------------------------------------------------------------------
      | Der Godsensor mit Sichtfeld Funktionsblock nimmt die Bewegungsrichtung des EGOs und Fzgs als Input und gibt Daten einer Distanz und Kollisionserkennung zurück.
      | -----------------------------------------------------------------------------------------------------------
      | Die Relevanz Kontrolle prüft, wie Relevant das Erkannte Fzg ist
  EGO Pos1 : Inport
  Fzg Pos Y : Inport  Port=2
  Kreuzung y : Inport  Port=3
  Kreuzung x : Inport  Port=4
  "God Sensor mit Sichtfeld " : MATLAB Function  TreatAsAtomicUnit=on
  Relevanz Kontrolle : Subsystem
  distance : Outport
  collision : Outport  Port=2
  relevanz : Outport  Port=3
  wires:
  EGO Pos1/1 -> Relevanz Kontrolle/1(EGO Pos), "God Sensor mit Sichtfeld "/1(xEGO)
  "God Sensor mit Sichtfeld "/2(collision) -> collision/1
  "God Sensor mit Sichtfeld "/1(distance) -> Relevanz Kontrolle/4(distance), distance/1
  Fzg Pos Y/1 -> Relevanz Kontrolle/2(Fzg Pos Y), "God Sensor mit Sichtfeld "/2(yFzg)
  Kreuzung y/1 -> Relevanz Kontrolle/3(Kreuzung y)
  Kreuzung x/1 -> Relevanz Kontrolle/5(Kreuzung x)
  Relevanz Kontrolle/1(relevanz) -> relevanz/1

== system FAS_Kreuzungswarner_Simulation_V1/Sensor B/Radar ==
  note: Radar
      | -----------------------------------------------------------------------------------------------------------
      | God Sensor mit Sichtfeld Funktionsblock mit der allgemeinen Relevanz Kontrolle
      | -----------------------------------------------------------------------------------------------------------
      | Der Godsensor mit Sichtfeld Funktionsblock nimmt die Bewegungsrichtung des EGOs und Fzgs als Input und gibt Daten einer Distanz und Kollisionserkennung zurück.
      | -----------------------------------------------------------------------------------------------------------
      | Die Relevanz Kontrolle prüft, wie Relevant das Erkannte Fzg ist
  EGO Pos1 : Inport
  Fzg Pos Y : Inport  Port=2
  Kreuzung y : Inport  Port=3
  Kreuzung x : Inport  Port=4
  God Sensor mit Sichtfeld 1 : MATLAB Function  TreatAsAtomicUnit=on
  Relevanz Kontrolle : Subsystem
  distance : Outport
  collision : Outport  Port=2
  relevanz : Outport  Port=3
  wires:
  EGO Pos1/1 -> God Sensor mit Sichtfeld 1/1(xEGO), Relevanz Kontrolle/1(EGO Pos)
  God Sensor mit Sichtfeld 1/2(collision) -> collision/1
  God Sensor mit Sichtfeld 1/1(distance) -> Relevanz Kontrolle/4(distance), distance/1
  Fzg Pos Y/1 -> God Sensor mit Sichtfeld 1/2(yFzg), Relevanz Kontrolle/2(Fzg Pos Y)
  Kreuzung y/1 -> Relevanz Kontrolle/3(Kreuzung y)
  Kreuzung x/1 -> Relevanz Kontrolle/5(Kreuzung x)
  Relevanz Kontrolle/1(relevanz) -> relevanz/1

== system FAS_Kreuzungswarner_Simulation_V1/Sensor B/Relevanz Kontrolle ==
  note: Gibt eine 1 aus wenn Fzg auf y Achse Fährt
      | Gibt eine -1 aus wenn Fzg auf x Achse Fährt
  xPos : Inport
  yPos : Inport  Port=2
  Bewegungs-Achse Fzg1 : MATLAB Function  TreatAsAtomicUnit=on
  Const -1 : Constant  Value=-1
  Const 1 : Constant
  Switch1 : Switch  Criteria=u2 > Threshold  Threshold=1  SaturateOnIntegerOverflow=off  InputSameDT=off
  Unit Delay4 : UnitDelay  SampleTime=-1  HasFrameUpgradeWarning=on
  Unit Delay5 : UnitDelay  SampleTime=-1  HasFrameUpgradeWarning=on
  relevanz1 : Outport
  wires:
  Const -1/1 -> Switch1/3
  Unit Delay4/1 -> Bewegungs-Achse Fzg1/2(xFzg_prev)
  yPos/1 -> Unit Delay5/1, Bewegungs-Achse Fzg1/3(yFzg)
  Unit Delay5/1 -> Bewegungs-Achse Fzg1/4(yFzg_prev)
  xPos/1 -> Unit Delay4/1, Bewegungs-Achse Fzg1/1(xFzg)
  Const 1/1 -> Switch1/1
  Switch1/1 -> relevanz1/1
  Bewegungs-Achse Fzg1/1(bewegung) -> Switch1/2

== system FAS_Kreuzungswarner_Simulation_V1/Sensor B/Umwandlung v in s ==
  note: Integrieren der Geschwindigkeit, um auf die Position zu kommen.
      | Davon wird dann die Startpos hinzugerechnet
  In1 : Inport
  Add : Sum
  Constant : Constant  Value=startPositionEGO
  Integrator : Integrator
  EGO Pos1 : Outport
  wires:
  Add/1 -> EGO Pos1/1
  Constant/1 -> Add/2
  Integrator/1 -> Add/1
  In1/1 -> Integrator/1

== system FAS_Kreuzungswarner_Simulation_V1/Sensor B/Umwandlung v in s1 ==
  note: Integrieren der Geschwindigkeit, um auf die Position zu kommen.
      | Davon wird dann die Startpos hinzugerechnet
  In1 : Inport
  Add : Sum
  Constant : Constant  Value=startPositionFzg
  Integrator : Integrator
  Fzg Pos : Outport
  wires:
  Add/1 -> Fzg Pos/1
  Constant/1 -> Add/2
  Integrator/1 -> Add/1
  In1/1 -> Integrator/1

== system FAS_Kreuzungswarner_Simulation_V1/Sensor B/Umwandlung v in s2 ==
  note: Integrieren der Geschwindigkeit, um auf die Position zu kommen.
      | Davon wird dann die Startpos hinzugerechnet
  In1 : Inport
  Add : Sum
  Constant : Constant  Value=startPositionFzg2
  Constant1 : Constant  Value=yEGO
  Integrator : Integrator
  Fzg xPos : Outport
  Fzg yPos1 : Outport  Port=2
  wires:
  Add/1 -> Fzg xPos/1
  Constant/1 -> Add/2
  Integrator/1 -> Add/1
  In1/1 -> Integrator/1
  Constant1/1 -> Fzg yPos1/1

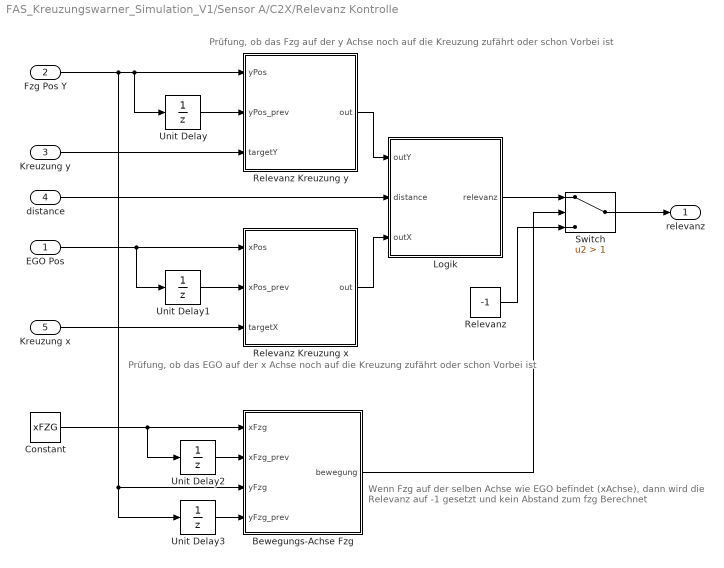
== system FAS_Kreuzungswarner_Simulation_V1/Sensor A/C2X/Relevanz Kontrolle ==
  note: Prüfung, ob das Fzg auf der y Achse noch auf die Kreuzung zufährt oder schon Vorbei ist
  note: Wenn Fzg auf der selben Achse wie EGO befindet (xAchse),
      | dann wird die Relevanz auf -1 gesetzt und kein Abstand zum fzg Berechnet
  note: Prüfung, ob das EGO auf der x Achse noch auf die Kreuzung zufährt oder schon Vorbei ist
  EGO Pos : Inport
  Fzg Pos Y : Inport  Port=2
  Kreuzung y : Inport  Port=3
  distance : Inport  Port=4
  Kreuzung x : Inport  Port=5
  Bewegungs-Achse Fzg : MATLAB Function  TreatAsAtomicUnit=on
  Constant : Constant  Value=xFZG
  Logik : MATLAB Function  TreatAsAtomicUnit=on
  Relevanz : Constant  Value=-1
  Relevanz Kreuzung x : MATLAB Function  TreatAsAtomicUnit=on
  Relevanz Kreuzung y : MATLAB Function  TreatAsAtomicUnit=on
  Switch : Switch  Criteria=u2 > Threshold  Threshold=1  SaturateOnIntegerOverflow=off  InputSameDT=off
  Unit Delay{,1..3} (4 alike) : UnitDelay  SampleTime=-1  HasFrameUpgradeWarning=on
  relevanz : Outport
  wires:
  Unit Delay/1 -> Relevanz Kreuzung y/2(yPos_prev)
  Fzg Pos Y/1 -> Unit Delay3/1, Bewegungs-Achse Fzg/3(yFzg), Unit Delay/1, Relevanz Kreuzung y/1(yPos)
  distance/1 -> Logik/2(distance)
  Kreuzung y/1 -> Relevanz Kreuzung y/3(targetY)
  Kreuzung x/1 -> Relevanz Kreuzung x/3(targetX)
  Unit Delay1/1 -> Relevanz Kreuzung x/2(xPos_prev)
  EGO Pos/1 -> Unit Delay1/1, Relevanz Kreuzung x/1(xPos)
  Relevanz Kreuzung x/1(out) -> Logik/3(outX)
  Relevanz Kreuzung y/1(out) -> Logik/1(outY)
  Unit Delay2/1 -> Bewegungs-Achse Fzg/2(xFzg_prev)
  Unit Delay3/1 -> Bewegungs-Achse Fzg/4(yFzg_prev)
  Constant/1 -> Unit Delay2/1, Bewegungs-Achse Fzg/1(xFzg)
  Bewegungs-Achse Fzg/1(bewegung) -> Switch/2
  Logik/1(relevanz) -> Switch/1
  Switch/1 -> relevanz/1
  Relevanz/1 -> Switch/3

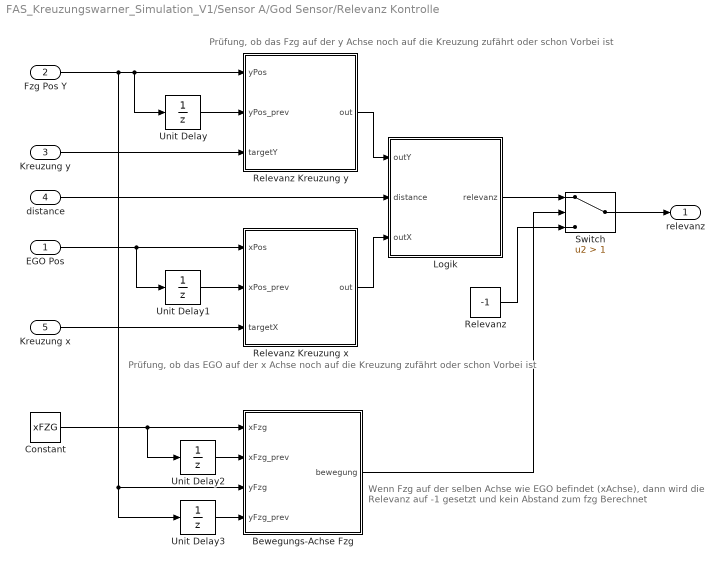
== system FAS_Kreuzungswarner_Simulation_V1/Sensor A/God Sensor/Relevanz Kontrolle ==
  note: Prüfung, ob das Fzg auf der y Achse noch auf die Kreuzung zufährt oder schon Vorbei ist
  note: Wenn Fzg auf der selben Achse wie EGO befindet (xAchse),
      | dann wird die Relevanz auf -1 gesetzt und kein Abstand zum fzg Berechnet
  note: Prüfung, ob das EGO auf der x Achse noch auf die Kreuzung zufährt oder schon Vorbei ist
  EGO Pos : Inport
  Fzg Pos Y : Inport  Port=2
  Kreuzung y : Inport  Port=3
  distance : Inport  Port=4
  Kreuzung x : Inport  Port=5
  Bewegungs-Achse Fzg : MATLAB Function  TreatAsAtomicUnit=on
  Constant : Constant  Value=xFZG
  Logik : MATLAB Function  TreatAsAtomicUnit=on
  Relevanz : Constant  Value=-1
  Relevanz Kreuzung x : MATLAB Function  TreatAsAtomicUnit=on
  Relevanz Kreuzung y : MATLAB Function  TreatAsAtomicUnit=on
  Switch : Switch  Criteria=u2 > Threshold  Threshold=1  SaturateOnIntegerOverflow=off  InputSameDT=off
  Unit Delay{,1..3} (4 alike) : UnitDelay  SampleTime=-1  HasFrameUpgradeWarning=on
  relevanz : Outport
  wires:
  Unit Delay/1 -> Relevanz Kreuzung y/2(yPos_prev)
  Fzg Pos Y/1 -> Unit Delay3/1, Bewegungs-Achse Fzg/3(yFzg), Unit Delay/1, Relevanz Kreuzung y/1(yPos)
  distance/1 -> Logik/2(distance)
  Kreuzung y/1 -> Relevanz Kreuzung y/3(targetY)
  Kreuzung x/1 -> Relevanz Kreuzung x/3(targetX)
  Unit Delay1/1 -> Relevanz Kreuzung x/2(xPos_prev)
  EGO Pos/1 -> Unit Delay1/1, Relevanz Kreuzung x/1(xPos)
  Relevanz Kreuzung x/1(out) -> Logik/3(outX)
  Relevanz Kreuzung y/1(out) -> Logik/1(outY)
  Unit Delay2/1 -> Bewegungs-Achse Fzg/2(xFzg_prev)
  Unit Delay3/1 -> Bewegungs-Achse Fzg/4(yFzg_prev)
  Constant/1 -> Unit Delay2/1, Bewegungs-Achse Fzg/1(xFzg)
  Bewegungs-Achse Fzg/1(bewegung) -> Switch/2
  Logik/1(relevanz) -> Switch/1
  Switch/1 -> relevanz/1
  Relevanz/1 -> Switch/3

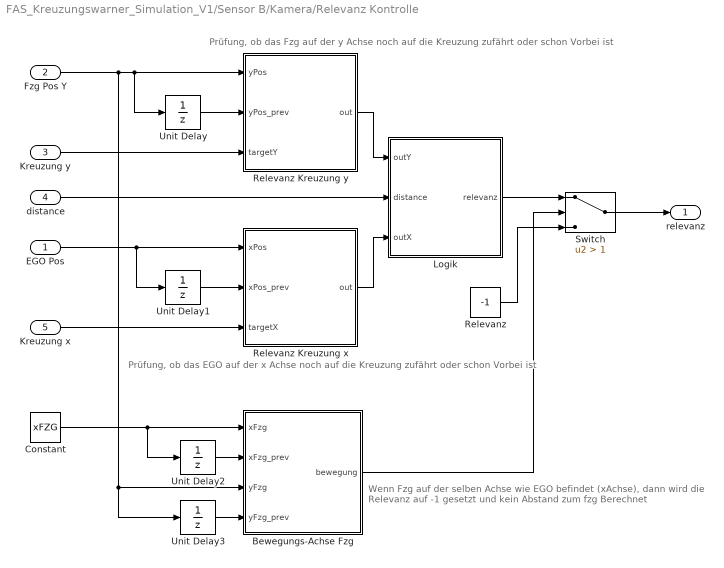
== system FAS_Kreuzungswarner_Simulation_V1/Sensor B/Kamera/Relevanz Kontrolle ==
  note: Prüfung, ob das Fzg auf der y Achse noch auf die Kreuzung zufährt oder schon Vorbei ist
  note: Wenn Fzg auf der selben Achse wie EGO befindet (xAchse),
      | dann wird die Relevanz auf -1 gesetzt und kein Abstand zum fzg Berechnet
  note: Prüfung, ob das EGO auf der x Achse noch auf die Kreuzung zufährt oder schon Vorbei ist
  EGO Pos : Inport
  Fzg Pos Y : Inport  Port=2
  Kreuzung y : Inport  Port=3
  distance : Inport  Port=4
  Kreuzung x : Inport  Port=5
  Bewegungs-Achse Fzg : MATLAB Function  TreatAsAtomicUnit=on
  Constant : Constant  Value=xFZG
  Logik : MATLAB Function  TreatAsAtomicUnit=on
  Relevanz : Constant  Value=-1
  Relevanz Kreuzung x : MATLAB Function  TreatAsAtomicUnit=on
  Relevanz Kreuzung y : MATLAB Function  TreatAsAtomicUnit=on
  Switch : Switch  Criteria=u2 > Threshold  Threshold=1  SaturateOnIntegerOverflow=off  InputSameDT=off
  Unit Delay{,1..3} (4 alike) : UnitDelay  SampleTime=-1  HasFrameUpgradeWarning=on
  relevanz : Outport
  wires:
  Unit Delay/1 -> Relevanz Kreuzung y/2(yPos_prev)
  Fzg Pos Y/1 -> Unit Delay3/1, Bewegungs-Achse Fzg/3(yFzg), Unit Delay/1, Relevanz Kreuzung y/1(yPos)
  distance/1 -> Logik/2(distance)
  Kreuzung y/1 -> Relevanz Kreuzung y/3(targetY)
  Kreuzung x/1 -> Relevanz Kreuzung x/3(targetX)
  Unit Delay1/1 -> Relevanz Kreuzung x/2(xPos_prev)
  EGO Pos/1 -> Unit Delay1/1, Relevanz Kreuzung x/1(xPos)
  Relevanz Kreuzung x/1(out) -> Logik/3(outX)
  Relevanz Kreuzung y/1(out) -> Logik/1(outY)
  Unit Delay2/1 -> Bewegungs-Achse Fzg/2(xFzg_prev)
  Unit Delay3/1 -> Bewegungs-Achse Fzg/4(yFzg_prev)
  Constant/1 -> Unit Delay2/1, Bewegungs-Achse Fzg/1(xFzg)
  Bewegungs-Achse Fzg/1(bewegung) -> Switch/2
  Logik/1(relevanz) -> Switch/1
  Switch/1 -> relevanz/1
  Relevanz/1 -> Switch/3

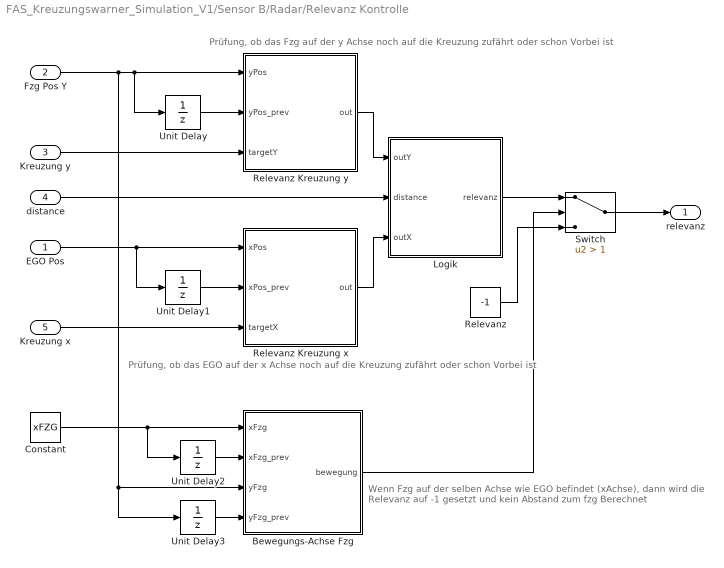
== system FAS_Kreuzungswarner_Simulation_V1/Sensor B/Radar/Relevanz Kontrolle ==
  note: Prüfung, ob das Fzg auf der y Achse noch auf die Kreuzung zufährt oder schon Vorbei ist
  note: Wenn Fzg auf der selben Achse wie EGO befindet (xAchse),
      | dann wird die Relevanz auf -1 gesetzt und kein Abstand zum fzg Berechnet
  note: Prüfung, ob das EGO auf der x Achse noch auf die Kreuzung zufährt oder schon Vorbei ist
  EGO Pos : Inport
  Fzg Pos Y : Inport  Port=2
  Kreuzung y : Inport  Port=3
  distance : Inport  Port=4
  Kreuzung x : Inport  Port=5
  Bewegungs-Achse Fzg : MATLAB Function  TreatAsAtomicUnit=on
  Constant : Constant  Value=xFZG
  Logik : MATLAB Function  TreatAsAtomicUnit=on
  Relevanz : Constant  Value=-1
  Relevanz Kreuzung x : MATLAB Function  TreatAsAtomicUnit=on
  Relevanz Kreuzung y : MATLAB Function  TreatAsAtomicUnit=on
  Switch : Switch  Criteria=u2 > Threshold  Threshold=1  SaturateOnIntegerOverflow=off  InputSameDT=off
  Unit Delay{,1..3} (4 alike) : UnitDelay  SampleTime=-1  HasFrameUpgradeWarning=on
  relevanz : Outport
  wires:
  Unit Delay/1 -> Relevanz Kreuzung y/2(yPos_prev)
  Fzg Pos Y/1 -> Unit Delay3/1, Bewegungs-Achse Fzg/3(yFzg), Unit Delay/1, Relevanz Kreuzung y/1(yPos)
  distance/1 -> Logik/2(distance)
  Kreuzung y/1 -> Relevanz Kreuzung y/3(targetY)
  Kreuzung x/1 -> Relevanz Kreuzung x/3(targetX)
  Unit Delay1/1 -> Relevanz Kreuzung x/2(xPos_prev)
  EGO Pos/1 -> Unit Delay1/1, Relevanz Kreuzung x/1(xPos)
  Relevanz Kreuzung x/1(out) -> Logik/3(outX)
  Relevanz Kreuzung y/1(out) -> Logik/1(outY)
  Unit Delay2/1 -> Bewegungs-Achse Fzg/2(xFzg_prev)
  Unit Delay3/1 -> Bewegungs-Achse Fzg/4(yFzg_prev)
  Constant/1 -> Unit Delay2/1, Bewegungs-Achse Fzg/1(xFzg)
  Bewegungs-Achse Fzg/1(bewegung) -> Switch/2
  Logik/1(relevanz) -> Switch/1
  Switch/1 -> relevanz/1
  Relevanz/1 -> Switch/3

== matlab function FAS_Kreuzungswarner_Simulation_V1/Sensor A/C2X/Fzg Vorhanden? ==
  data: u input; y output
function y = check_signal(u)
    if isnan(u)  % Prüft, ob das Signal NaN ist
        y = 0;   % Kein Signal vorhanden
    else
        y = 1;   % Signal ist vorhanden
    end
end

== matlab function FAS_Kreuzungswarner_Simulation_V1/Sensor A/God Sensor/Relevanz Kontrolle/Logik ==
  data: outY input; distance input; outX input; relevanz output; defaultDistance parameter
function relevanz = direction(outY, distance, outX, defaultDistance)
% Wenn der Sensor ein fzg erkennt (distance < defaultDistance) Wir wenn
% EGO und Fzg noch vor der Kreuzung sind eine Relevanz ausgegeben (1). Wenn
% nicht wird das Fzg als nicht Relevant gemarkt (-1)

    if distance < defaultDistance 
        if outX == 1 && outY == 1
            relevanz = 1;
        else
            relevanz = -1;
        end
    else
        relevanz = 0;
    end

end
